simulink model "merged"  (R2024b)
settings: Solver=VariableStepAuto  StartTime=0.0  StopTime=10.0  RelTol=1e-3
libraries: simulink_extras x1
settings Model: PacingRate=0.450000  Creator=Reon Dsouze  LastModifiedBy=Reon Dsouze

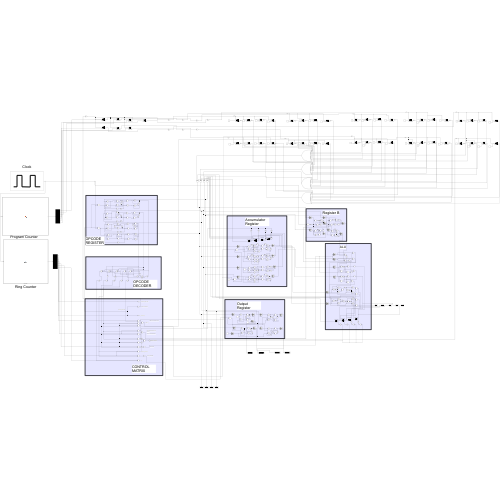
[thumbnail: Simulink's stored preview of the top-level diagram]
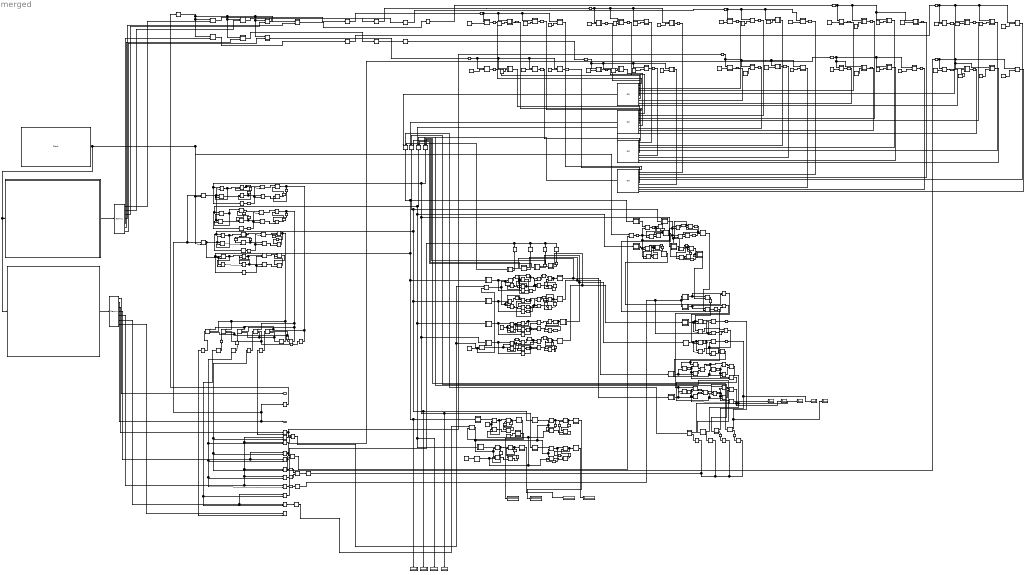
== system merged ==
  note: Clock
  note: Ring Counter
  note: Program Counter
  note: Register B
  note: ALU
  note: Output Register
  note: Accumulator Register
  note: Increment Program Counter
  note: CONTROL MATRIX
  note: enable A reg to data bus
  note: enable subtract
  note: enable sub to data bus from mem
  note: OPCODE DECODER
  note: enable ALU to data bus
  note: enable add to data bus from mem
  note: load A reg
  note: enable load a to data bus from mem
  note: load B reg
  note: halt
  note: Enable mmr to data bus
  note: Opcode reg latches data
  note: grnd mem disp
  note: output reg latches data
  note: OPCODE
      | REGISTER
  AND{,1..9} (10 alike) : Logic  IconShape=distinctive  AllPortsSameDT=off  OutDataTypeStr=boolean
  Clock1 : simulink_extras/Flip Flops/Clock  period=2
  Constant{,1..44} (45 alike) : Constant
  Delay{,1..84} (85 alike) : Delay
  Demux : Demux  Outputs=7
  Demux1 : Demux  Outputs=7
  Display{,1..12} (13 alike) : Display
  NAND{,1..52,54..56,58..60,62..64,66..107,113..120,122..132} (123 alike) : Logic  Operator=NAND  IconShape=distinctive  AllPortsSameDT=off  OutDataTypeStr=boolean
  NAND{53,57,61,65,108..112,121} (10 alike) : Logic  Operator=NAND  Inputs=3  IconShape=distinctive  AllPortsSameDT=off  OutDataTypeStr=boolean
  NOT{,1..72} (73 alike) : Logic  Operator=NOT  IconShape=distinctive  AllPortsSameDT=off  OutDataTypeStr=boolean
  OR : Logic  Operator=OR  IconShape=distinctive  AllPortsSameDT=off  OutDataTypeStr=boolean
  OR1 : Logic  Operator=OR  IconShape=distinctive  AllPortsSameDT=off  OutDataTypeStr=boolean
  OR{2..5} (4 alike) : Logic  Operator=OR  Inputs=3  IconShape=distinctive  AllPortsSameDT=off  OutDataTypeStr=boolean
  OR{6..9} (4 alike) : Logic  Operator=OR  Inputs=10  IconShape=distinctive  AllPortsSameDT=off  OutDataTypeStr=boolean
  Program Counter : MATLAB Function  TreatAsAtomicUnit=on
  Ring Counter : MATLAB Function  TreatAsAtomicUnit=on
  Tri state buffer : Subsystem
      mask Display:
      | % Draw the triangle
      | patch([1 0 1], [0 0.5 1], [0 0 0])  % Left-pointing triangle
  Tri state buffer1 : Subsystem
      mask Display:
      | % Draw the triangle
      | patch([1 0 1], [0 0.5 1], [0 0 0])  % Left-pointing triangle
  Tri state buffer10 : Subsystem
      mask Display:
      | % Draw the triangle
      | patch([1 0 1], [0 0.5 1], [0 0 0])  % Left-pointing triangle
  Tri state buffer11 : Subsystem
      mask Display:
      | % Draw the triangle
      | patch([1 0 1], [0 0.5 1], [0 0 0])  % Left-pointing triangle
  Tri state buffer12 : Subsystem
      mask Display:
      | % Draw the triangle
      | patch([1 0 1], [0 0.5 1], [0 0 0])  % Left-pointing triangle
  Tri state buffer13 : Subsystem
      mask Display:
      | % Draw the triangle
      | patch([1 0 1], [0 0.5 1], [0 0 0])  % Left-pointing triangle
  Tri state buffer14 : Subsystem
      mask Display:
      | % Draw the triangle
      | patch([1 0 1], [0 0.5 1], [0 0 0])  % Left-pointing triangle
  Tri state buffer15 : Subsystem
      mask Display:
      | % Draw the triangle
      | patch([1 0 1], [0 0.5 1], [0 0 0])  % Left-pointing triangle
  Tri state buffer16 : Subsystem
      mask Display:
      | % Draw the triangle
      | patch([1 0 1], [0 0.5 1], [0 0 0])  % Left-pointing triangle
  Tri state buffer17 : Subsystem
      mask Display:
      | % Draw the triangle
      | patch([1 0 1], [0 0.5 1], [0 0 0])  % Left-pointing triangle
  Tri state buffer18 : Subsystem
      mask Display:
      | % Draw the triangle
      | patch([1 0 1], [0 0.5 1], [0 0 0])  % Left-pointing triangle
  Tri state buffer19 : Subsystem
      mask Display:
      | % Draw the triangle
      | patch([1 0 1], [0 0.5 1], [0 0 0])  % Left-pointing triangle
  Tri state buffer2 : Subsystem
      mask Display:
      | % Draw the triangle
      | patch([1 0 1], [0 0.5 1], [0 0 0])  % Left-pointing triangle
  Tri state buffer20 : Subsystem
      mask Display:
      | % Draw the triangle
      | patch([1 0 1], [0 0.5 1], [0 0 0])  % Left-pointing triangle
  Tri state buffer21 : Subsystem
      mask Display:
      | % Draw the triangle
      | patch([1 0 1], [0 0.5 1], [0 0 0])  % Left-pointing triangle
  Tri state buffer22 : Subsystem
      mask Display:
      | % Draw the triangle
      | patch([1 0 1], [0 0.5 1], [0 0 0])  % Left-pointing triangle
  Tri state buffer23 : Subsystem
      mask Display:
      | % Draw the triangle
      | patch([1 0 1], [0 0.5 1], [0 0 0])  % Left-pointing triangle
  Tri state buffer24 : Subsystem
      mask Display:
      | % Draw the triangle
      | patch([1 0 1], [0 0.5 1], [0 0 0])  % Left-pointing triangle
  Tri state buffer25 : Subsystem
      mask Display:
      | % Draw the triangle
      | patch([1 0 1], [0 0.5 1], [0 0 0])  % Left-pointing triangle
  Tri state buffer26 : Subsystem
      mask Display:
      | % Draw the triangle
      | patch([1 0 1], [0 0.5 1], [0 0 0])  % Left-pointing triangle
  Tri state buffer27 : Subsystem
      mask Display:
      | % Draw the triangle
      | patch([1 0 1], [0 0.5 1], [0 0 0])  % Left-pointing triangle
  Tri state buffer28 : Subsystem
      mask Display:
      | % Draw the triangle
      | patch([1 0 1], [0 0.5 1], [0 0 0])  % Left-pointing triangle
  Tri state buffer29 : Subsystem
      mask Display:
      | % Draw the triangle
      | patch([1 0 1], [0 0.5 1], [0 0 0])  % Left-pointing triangle
  Tri state buffer3 : Subsystem
      mask Display:
      | % Draw the triangle
      | patch([1 0 1], [0 0.5 1], [0 0 0])  % Left-pointing triangle
  Tri state buffer30 : Subsystem
      mask Display:
      | % Draw the triangle
      | patch([1 0 1], [0 0.5 1], [0 0 0])  % Left-pointing triangle
  Tri state buffer31 : Subsystem
      mask Display:
      | % Draw the triangle
      | patch([1 0 1], [0 0.5 1], [0 0 0])  % Left-pointing triangle
  Tri state buffer32 : Subsystem
      mask Display:
      | % Draw the triangle
      | patch([1 0 1], [0 0.5 1], [0 0 0])  % Left-pointing triangle
  Tri state buffer33 : Subsystem
      mask Display:
      | % Draw the triangle
      | patch([1 0 1], [0 0.5 1], [0 0 0])  % Left-pointing triangle
  Tri state buffer34 : Subsystem
      mask Display:
      | % Draw the triangle
      | patch([1 0 1], [0 0.5 1], [0 0 0])  % Left-pointing triangle
  Tri state buffer35 : Subsystem
      mask Display:
      | % Draw the triangle
      | patch([1 0 1], [0 0.5 1], [0 0 0])  % Left-pointing triangle
  Tri state buffer36 : Subsystem
      mask Display:
      | % Draw the triangle
      | patch([1 0 1], [0 0.5 1], [0 0 0])  % Left-pointing triangle
  Tri state buffer37 : Subsystem
      mask Display:
      | % Draw the triangle
      | patch([1 0 1], [0 0.5 1], [0 0 0])  % Left-pointing triangle
  Tri state buffer38 : Subsystem
      mask Display:
      | % Draw the triangle
      | patch([1 0 1], [0 0.5 1], [0 0 0])  % Left-pointing triangle
  Tri state buffer39 : Subsystem
      mask Display:
      | % Draw the triangle
      | patch([1 0 1], [0 0.5 1], [0 0 0])  % Left-pointing triangle
  Tri state buffer4 : Subsystem
      mask Display:
      | % Draw the triangle
      | patch([1 0 1], [0 0.5 1], [0 0 0])  % Left-pointing triangle
  Tri state buffer40 : Subsystem
      mask Display:
      | % Draw the triangle
      | patch([1 0 1], [0 0.5 1], [0 0 0])  % Left-pointing triangle
  Tri state buffer41 : Subsystem
      mask Display:
      | % Draw the triangle
      | patch([1 0 1], [0 0.5 1], [0 0 0])  % Left-pointing triangle
  Tri state buffer42 : Subsystem
      mask Display:
      | % Draw the triangle
      | patch([1 0 1], [0 0.5 1], [0 0 0])  % Left-pointing triangle
  Tri state buffer43 : Subsystem
      mask Display:
      | % Draw the triangle
      | patch([1 0 1], [0 0.5 1], [0 0 0])  % Left-pointing triangle
  Tri state buffer44 : Subsystem
      mask Display:
      | % Draw the triangle
      | patch([1 0 1], [0 0.5 1], [0 0 0])  % Left-pointing triangle
  Tri state buffer45 : Subsystem
      mask Display:
      | % Draw the triangle
      | patch([1 0 1], [0 0.5 1], [0 0 0])  % Left-pointing triangle
  Tri state buffer46 : Subsystem
      mask Display:
      | % Draw the triangle
      | patch([1 0 1], [0 0.5 1], [0 0 0])  % Left-pointing triangle
  Tri state buffer47 : Subsystem
      mask Display:
      | % Draw the triangle
      | patch([1 0 1], [0 0.5 1], [0 0 0])  % Left-pointing triangle
  Tri state buffer48 : Subsystem
      mask Display:
      | % Draw the triangle
      | patch([1 0 1], [0 0.5 1], [0 0 0])  % Left-pointing triangle
  Tri state buffer49 : Subsystem
      mask Display:
      | % Draw the triangle
      | patch([1 0 1], [0 0.5 1], [0 0 0])  % Left-pointing triangle
  Tri state buffer5 : Subsystem
      mask Display:
      | % Draw the triangle
      | patch([1 0 1], [0 0.5 1], [0 0 0])  % Left-pointing triangle
  Tri state buffer50 : Subsystem
      mask Display:
      | % Draw the triangle
      | patch([1 0 1], [0 0.5 1], [0 0 0])  % Left-pointing triangle
  Tri state buffer51 : Subsystem
      mask Display:
      | % Draw the triangle
      | patch([1 0 1], [0 0.5 1], [0 0 0])  % Left-pointing triangle
  Tri state buffer52 : Subsystem
      mask Display:
      | % Draw the triangle
      | patch([1 0 1], [0 0.5 1], [0 0 0])  % Left-pointing triangle
  Tri state buffer53 : Subsystem
      mask Display:
      | % Draw the triangle
      | patch([1 0 1], [0 0.5 1], [0 0 0])  % Left-pointing triangle
  Tri state buffer54 : Subsystem
      mask Display:
      | % Draw the triangle
      | patch([1 0 1], [0 0.5 1], [0 0 0])  % Left-pointing triangle
  Tri state buffer55 : Subsystem
      mask Display:
      | % Draw the triangle
      | patch([1 0 1], [0 0.5 1], [0 0 0])  % Left-pointing triangle
  Tri state buffer6 : Subsystem
      mask Display:
      | % Draw the triangle
      | patch([1 0 1], [0 0.5 1], [0 0 0])  % Left-pointing triangle
  Tri state buffer8 : Subsystem
      mask Display:
      | % Draw the triangle
      | patch([1 0 1], [0 0.5 1], [0 0 0])  % Left-pointing triangle
  Tri state buffer9 : Subsystem
      mask Display:
      | % Draw the triangle
      | patch([1 0 1], [0 0.5 1], [0 0 0])  % Left-pointing triangle
  XOR{,1..7} (8 alike) : Logic  Operator=XOR  IconShape=distinctive  AllPortsSameDT=off  OutDataTypeStr=boolean
  buffer : Subsystem
      mask Display: patch([0 1 0], [0 0.5 1], [0.5 0.5 0.5]);  % This draws a triangle
  buffer1 : Subsystem
      mask Display: patch([0 1 0], [0 0.5 1], [0.5 0.5 0.5]);  % This draws a triangle
  buffer10 : Subsystem
      mask Display: patch([0 1 0], [0 0.5 1], [0.5 0.5 0.5]);  % This draws a triangle
  buffer11 : Subsystem
      mask Display: patch([0 1 0], [0 0.5 1], [0.5 0.5 0.5]);  % This draws a triangle
  buffer12 : Subsystem
      mask Display: patch([0 1 0], [0 0.5 1], [0.5 0.5 0.5]);  % This draws a triangle
  buffer13 : Subsystem
      mask Display: patch([0 1 0], [0 0.5 1], [0.5 0.5 0.5]);  % This draws a triangle
  buffer14 : Subsystem
      mask Display: patch([0 1 0], [0 0.5 1], [0.5 0.5 0.5]);  % This draws a triangle
  buffer15 : Subsystem
      mask Display: patch([0 1 0], [0 0.5 1], [0.5 0.5 0.5]);  % This draws a triangle
  buffer16 : Subsystem
      mask Display: patch([0 1 0], [0 0.5 1], [0.5 0.5 0.5]);  % This draws a triangle
  buffer17 : Subsystem
      mask Display: patch([0 1 0], [0 0.5 1], [0.5 0.5 0.5]);  % This draws a triangle
  buffer18 : Subsystem
      mask Display: patch([0 1 0], [0 0.5 1], [0.5 0.5 0.5]);  % This draws a triangle
  buffer19 : Subsystem
      mask Display: patch([0 1 0], [0 0.5 1], [0.5 0.5 0.5]);  % This draws a triangle
  buffer2 : Subsystem
      mask Display: patch([0 1 0], [0 0.5 1], [0.5 0.5 0.5]);  % This draws a triangle
  buffer20 : Subsystem
      mask Display: patch([0 1 0], [0 0.5 1], [0.5 0.5 0.5]);  % This draws a triangle
  buffer21 : Subsystem
      mask Display: patch([0 1 0], [0 0.5 1], [0.5 0.5 0.5]);  % This draws a triangle
  buffer22 : Subsystem
      mask Display: patch([0 1 0], [0 0.5 1], [0.5 0.5 0.5]);  % This draws a triangle
  buffer23 : Subsystem
      mask Display: patch([0 1 0], [0 0.5 1], [0.5 0.5 0.5]);  % This draws a triangle
  buffer24 : Subsystem
      mask Display: patch([0 1 0], [0 0.5 1], [0.5 0.5 0.5]);  % This draws a triangle
  buffer25 : Subsystem
      mask Display: patch([0 1 0], [0 0.5 1], [0.5 0.5 0.5]);  % This draws a triangle
  buffer26 : Subsystem
      mask Display: patch([0 1 0], [0 0.5 1], [0.5 0.5 0.5]);  % This draws a triangle
  buffer27 : Subsystem
      mask Display: patch([0 1 0], [0 0.5 1], [0.5 0.5 0.5]);  % This draws a triangle
  buffer28 : Subsystem
      mask Display: patch([0 1 0], [0 0.5 1], [0.5 0.5 0.5]);  % This draws a triangle
  buffer29 : Subsystem
      mask Display: patch([0 1 0], [0 0.5 1], [0.5 0.5 0.5]);  % This draws a triangle
  buffer3 : Subsystem
      mask Display: patch([0 1 0], [0 0.5 1], [0.5 0.5 0.5]);  % This draws a triangle
  buffer30 : Subsystem
      mask Display: patch([0 1 0], [0 0.5 1], [0.5 0.5 0.5]);  % This draws a triangle
  buffer31 : Subsystem
      mask Display: patch([0 1 0], [0 0.5 1], [0.5 0.5 0.5]);  % This draws a triangle
  buffer4 : Subsystem
      mask Display: patch([0 1 0], [0 0.5 1], [0.5 0.5 0.5]);  % This draws a triangle
  buffer5 : Subsystem
      mask Display: patch([0 1 0], [0 0.5 1], [0.5 0.5 0.5]);  % This draws a triangle
  buffer6 : Subsystem
      mask Display: patch([0 1 0], [0 0.5 1], [0.5 0.5 0.5]);  % This draws a triangle
  buffer7 : Subsystem
      mask Display: patch([0 1 0], [0 0.5 1], [0.5 0.5 0.5]);  % This draws a triangle
  buffer8 : Subsystem
      mask Display: patch([0 1 0], [0 0.5 1], [0.5 0.5 0.5]);  % This draws a triangle
  buffer9 : Subsystem
      mask Display: patch([0 1 0], [0 0.5 1], [0.5 0.5 0.5]);  % This draws a triangle
  Out2 : Outport
  Out3 : Outport  Port=2
  wires:
  buffer15/1(Out1) -> Tri state buffer6/1(In1), buffer5/1(In1)
  NAND80/1 -> NAND79/2
  buffer5/1(Out1) -> NAND9/2, NAND11/2
  NAND76/1 -> NAND75/2
  NAND75/1 -> NAND77/2
  NAND21/1 -> Delay35/1, buffer15/1(In1)
  NAND59/1 -> Delay54/1, buffer27/1(In1)
  NAND7/1 -> Display10/1, Tri state buffer2/1(In1)
  AND1/1 -> Delay78/1
  NAND39/1 -> NAND41/2
  NAND67/1 -> NAND69/2
  Constant2/1 -> NAND50/2, NAND53/1
  XOR5/1 -> Delay67/1
  buffer4/1(Out1) -> NAND/2, NAND2/2
  NAND31/1 -> NAND33/2
  NAND58/1 -> NAND59/1, Delay56/1
  NAND72/1 -> NAND71/2
  NAND63/1 -> Delay57/1, buffer30/1(In1)
  NOT6/1 -> Delay70/1
  NAND45/1 -> Delay19/1, buffer21/1(In1)
  NAND23/1 -> NAND24/2
  NOT7/1 -> Delay66/1
  NOT2/1 -> NAND34/2, NAND35/1
  NAND1/1 -> NAND3/1
  NAND53/1 -> NAND52/2
  buffer1/1(Out1) -> XOR1/1, XOR3/1
  NAND55/1 -> buffer25/1(In1), Delay52/1
  NAND34/1 -> NAND37/1
  Constant1/1 -> AND5/2, AND6/2
  NAND15/1 -> NAND16/2
  buffer14/1(Out1) -> NAND30/1, NOT/1
  buffer7/1(Out1) -> NAND70/1
  NAND6/1 -> NAND7/2
  NAND62/1 -> Delay59/1, NAND63/1
  buffer10/1(Out1) -> XOR3/2
  buffer3/1(Out1) -> AND2/2, XOR6/2
  OR1/1 -> NAND6/2, NAND4/2
  NAND65/1 -> NAND64/2
  OR/1 -> AND3/2, XOR7/2
  buffer20/1(Out1) -> NAND46/1, NOT3/1
  NAND8/1 -> NAND15/2, NAND13/2
  NAND19/1 -> NAND20/2
  NAND2/1 -> NAND3/2
  Constant/1 -> NAND39/1, NAND38/2
  buffer8/1(Out1) -> NAND74/1
  XOR3/1 -> NAND9/1, NAND10/1
  NAND46/1 -> Delay17/1, NAND47/2
  NAND51/1 -> Delay46/1, buffer23/1(In1)
  AND7/1 -> NAND62/2, NAND65/1, NAND57/1, NAND54/2, NAND58/2, NAND61/1
  AND5/1 -> NAND27/1, NAND26/2, NAND31/1, NAND30/2
  XOR/1 -> Delay79/1
  NOT5/1 -> Tri state buffer5/2(In2)
  NAND16/1 -> Display9/1, Tri state buffer3/1(In1)
  NAND27/1 -> NAND29/2
  buffer22/1(Out1) -> NAND50/1
  buffer/1(Out1) -> XOR2/1, XOR/1
  NAND81/1 -> Delay14/1, buffer13/1(In1)
  buffer26/1(Out1) -> NAND58/1
  buffer18/1(Out1) -> NAND38/1, NOT2/1
  AND/1 -> OR/1
  NAND38/1 -> NAND39/2, NAND40/1
  buffer29/1(Out1) -> NAND62/1
  XOR6/1 -> Delay80/1
  NAND35/1 -> NAND36/2
  XOR2/1 -> AND2/1, XOR6/1
  buffer6/1(Out1) -> NAND66/1
  buffer11/1(Out1) -> XOR2/2
  buffer28/1(Out1) -> NAND57/3, NAND53/3, NAND65/3, NAND61/3
  NAND50/1 -> NAND53/2, NAND51/1
  NAND5/1 -> NAND7/1
  XOR7/1 -> Delay71/1
  NAND33/1 -> NAND32/2, NAND19/2
  buffer19/1(Out1) -> Tri state buffer4/1(In1), buffer3/1(In1)
  NAND54/1 -> Delay53/1, NAND55/1
  NAND25/1 -> Delay31/1, buffer17/1(In1)
  buffer13/1(Out1) -> XOR/2
  buffer9/1(Out1) -> NAND78/1
  buffer24/1(Out1) -> NAND54/1
  AND6/1 -> NAND46/2, NAND47/1
  AND4/1 -> Delay21/1
  NOT3/1 -> NAND42/2, NAND43/1
  NAND47/1 -> NAND49/2
  buffer16/1(Out1) -> NAND26/1, NOT1/1
  NOT4/1 -> Tri state buffer6/2(In2)
  NAND14/1 -> NAND16/1
  NAND40/1 -> NAND41/1, NAND34/1
  NAND57/1 -> NAND56/2
  NAND43/1 -> NAND44/2
  AND3/1 -> OR1/2
  AND2/1 -> OR1/1
  buffer31/1(Out1) -> AND7/2
  buffer21/1(Out1) -> Tri state buffer52/1(In1), buffer2/1(In1)
  NAND68/1 -> NAND67/2
  buffer2/1(Out1) -> AND/2, XOR4/2
  buffer12/1(Out1) -> XOR1/2
  XOR4/1 -> Delay77/1
  NAND61/1 -> NAND60/2
  buffer17/1(Out1) -> Tri state buffer5/1(In1), buffer4/1(In1)
  NAND105/1 -> Delay/1, NAND127/1
  Demux1/3 -> NAND113/1
  Demux1/5 -> NAND126/1, NAND125/1, NAND120/1, NAND114/1, NAND115/1
  Demux1/1 -> Out3/1
  NOT22/1 -> NAND113/2
  NAND109/1 -> Delay76/1
  NAND103/1 -> NAND107/1
  NOT10/1 -> Delay74/1
  NAND108/1 -> NOT18/1
  NAND85/1 -> Delay4/1, NAND87/1
  NAND110/1 -> Delay84/1
  NAND100/1 -> NAND102/2
  NAND90/1 -> NAND91/2, NAND92/1
  OR4/1 -> NOT9/1, NAND131/1, buffer8/1(In1), Display6/1, buffer26/1(In1), buffer18/1(In1)
  NAND94/1 -> Delay1/1, NAND116/1
  NAND101/1 -> NAND102/1, NAND103/1
  NAND91/1 -> NAND93/2
  NOT9/1 -> Delay69/1
  NAND114/1 -> NAND121/2
  OR2/1 -> buffer6/1(In1), NOT17/1, NAND99/1, Display4/1, buffer22/1(In1), buffer14/1(In1)
  NOT18/1 -> NAND119/2
  NAND86/1 -> NAND89/1
  NOT17/1 -> NAND104/2, NAND103/2
  NAND130/1 -> Delay3/1, NOT11/1, NAND108/1, NAND110/1, NAND112/1
  NAND115/1 -> Delay81/1
  AND9/1 -> NAND91/1, NAND90/2, NAND100/1, NAND99/2
  NAND89/1 -> Delay7/1, NAND110/2, NOT10/1, NAND111/1
  NAND104/1 -> NAND106/2
  NAND123/1 -> NOT72/1, NAND124/2
  Ring Counter/1(y) -> Demux1/1
  Demux1/7 -> NAND119/1
  NAND128/1 -> NOT12/1
  NAND95/1 -> NAND98/1
  NOT11/1 -> Delay75/1
  Demux1/4 -> NAND122/1, NAND123/1
  NAND132/1 -> NAND85/2
  NOT23/1 -> NAND110/3, NAND111/3, NAND112/3
  NAND82/1 -> NAND83/2, NAND94/1
  Demux1/2 -> Out2/1, AND9/1, AND8/1, NOT15/1
  NOT8/1 -> Delay65/1
  NAND112/1 -> NOT22/1
  NAND107/1 -> NAND106/1
  NAND83/1 -> NAND105/2
  NAND98/1 -> Delay10/1, NAND108/2, NAND109/1, NOT23/1
  NOT20/1 -> NAND115/2, NAND126/2, NAND123/2, NAND120/2
  NAND93/1 -> Delay8/1, NAND96/1
  NAND84/1 -> Delay5/1, NAND86/1
  NAND92/1 -> Delay9/1, NAND95/1
  Demux1/6 -> NAND117/1, NAND118/1
  OR3/1 -> buffer7/1(In1), Display5/1, buffer24/1(In1), buffer16/1(In1), NOT16/1, NAND90/1
  NAND122/1 -> NOT71/1, NAND124/1
  NAND102/1 -> NAND104/1, NAND101/2
  Clock1/1 -> AND4/1, AND9/2, AND8/2, Ring Counter/1(clk), Program Counter/1(clk)
  NOT19/1 -> NAND118/2, NAND117/2
  NAND113/1 -> NOT70/1, NAND121/1
  NOT21/1 -> NAND125/2, NAND122/2, NAND114/2
  NAND99/1 -> NAND100/2, NAND101/1
  NOT16/1 -> Delay73/1
  NAND96/1 -> NAND97/2
  Program Counter/1(y) -> Demux/1
  NAND118/1 -> NOT14/1
  OR5/1 -> buffer9/1(In1), Display7/1, buffer29/1(In1), buffer20/1(In1), NOT8/1, NAND82/1
  NAND126/1 -> Delay82/1
  NAND120/1 -> NAND121/3
  AND8/1 -> NAND131/2, NAND132/1, NAND83/1, NAND82/2
  NAND125/1 -> Delay83/1
  NAND111/1 -> NOT21/1
  NAND127/1 -> NAND129/2
  NAND106/1 -> NAND107/2
  NAND116/1 -> NAND130/1
  NAND131/1 -> NAND132/2, NAND84/1
  NAND87/1 -> NAND88/2
  NOT24/1 -> Tri state buffer3/2(In2)
  NOT25/1 -> Tri state buffer2/2(In2)
  NOT26/1 -> Delay72/1
  NOT27/1 -> Delay68/1
  NOT12/1 -> NOT25/1, NOT26/1, NOT27/1, NOT24/1
  NOT13/1 -> XOR5/2, AND1/2, buffer1/1(In1), buffer/1(In1)
  NOT14/1 -> AND7/1
  NAND121/1 -> AND6/1, AND5/1
  Constant3/1 -> buffer28/1(In1)
  Tri state buffer3/1(Out1) -> OR2/2
  Tri state buffer2/1(Out1) -> OR3/2
  Tri state buffer1/1(Out1) -> OR4/2
  Tri state buffer/1(Out1) -> OR5/2
  Tri state buffer6/1(Out1) -> OR2/3
  Tri state buffer5/1(Out1) -> OR3/3
  Tri state buffer4/1(Out1) -> OR4/3
  Tri state buffer52/1(Out1) -> OR5/3
  Tri state buffer13/1(Out1) -> OR8/2
  Tri state buffer38/1(Out1) -> OR8/9
  Tri state buffer43/1(Out1) -> OR9/8
  Tri state buffer34/1(Out1) -> OR9/7
  Tri state buffer31/1(Out1) -> OR7/7
  Tri state buffer47/1(Out1) -> OR9/10
  Tri state buffer19/1(Out1) -> OR8/4
  Tri state buffer17/1(Out1) -> OR8/3
  Tri state buffer25/1(Out1) -> OR8/5
  Tri state buffer45/1(Out1) -> OR8/10
  Tri state buffer27/1(Out1) -> OR9/5
  Tri state buffer28/1(Out1) -> OR7/6
  Tri state buffer42/1(Out1) -> NOT56/1
  Tri state buffer39/1(Out1) -> NOT53/1
  NOT36/1 -> Tri state buffer20/1(In1), Tri state buffer18/1(In1), Tri state buffer21/1(In1), Tri state buffer19/1(In1)
  Tri state buffer16/1(Out1) -> NOT43/1
  NOT31/1 -> Tri state buffer14/1(In1), Tri state buffer12/1(In1), Tri state buffer15/1(In1), Tri state buffer13/1(In1)
  Tri state buffer51/1(Out1) -> NOT29/1
  Tri state buffer54/1(Out1) -> NOT55/1
  Tri state buffer32/1(Out1) -> NOT49/1
  Tri state buffer33/1(Out1) -> NOT50/1
  NOT28/1 -> Tri state buffer54/1(In1), Tri state buffer8/1(In1), Tri state buffer50/1(In1), Tri state buffer30/1(In1), Tri state buffer9/1(In1), Tri state buffer51/1(In1), Tri state buffer41/1(In1)
  Tri state buffer22/1(Out1) -> NOT42/1
  Tri state buffer48/1(Out1) -> NOT47/1
  Tri state buffer36/1(Out1) -> NOT51/1
  Tri state buffer23/1(Out1) -> NOT37/1
  NOT65/1 -> Tri state buffer33/1(In1), Tri state buffer31/1(In1), Tri state buffer34/1(In1), Tri state buffer32/1(In1)
  Tri state buffer18/1(Out1) -> NOT41/1
  Tri state buffer35/1(Out1) -> NOT57/1
  NOT32/1 -> Tri state buffer22/1(In1), Tri state buffer16/1(In1), Tri state buffer23/1(In1), Tri state buffer17/1(In1)
  Tri state buffer30/1(Out1) -> NOT39/1
  NOT63/1 -> NOT62/1
  Tri state buffer50/1(Out1) -> NOT48/1
  Tri state buffer44/1(Out1) -> NOT59/1
  Tri state buffer10/1(Out1) -> NOT69/1
  Tri state buffer41/1(Out1) -> NOT63/1
  Tri state buffer24/1(Out1) -> NOT45/1
  NOT66/1 -> NOT64/1
  Tri state buffer9/1(Out1) -> NOT66/1
  Tri state buffer14/1(Out1) -> NOT34/1
  Tri state buffer12/1(Out1) -> NOT35/1
  Tri state buffer21/1(Out1) -> NOT38/1
  NOT39/1 -> NOT31/1
  Tri state buffer8/1(Out1) -> NOT67/1
  Tri state buffer46/1(Out1) -> NOT58/1
  NOT61/1 -> Tri state buffer49/1(In1), Tri state buffer10/1(In1), Tri state buffer53/1(In1), Tri state buffer11/1(In1)
  Tri state buffer11/1(Out1) -> NOT30/1
  Tri state buffer37/1(Out1) -> NOT54/1
  Tri state buffer55/1(Out1) -> NOT60/1
  NOT29/1 -> NOT61/1
  Tri state buffer49/1(Out1) -> NOT68/1
  NOT67/1 -> NOT65/1
  NOT62/1 -> Tri state buffer26/1(In1), Tri state buffer24/1(In1), Tri state buffer27/1(In1), Tri state buffer25/1(In1)
  NOT48/1 -> NOT32/1
  Tri state buffer29/1(Out1) -> NOT46/1
  Tri state buffer40/1(Out1) -> NOT52/1
  NOT64/1 -> Tri state buffer55/1(In1), Tri state buffer28/1(In1), Tri state buffer48/1(In1), Tri state buffer29/1(In1)
  Tri state buffer15/1(Out1) -> NOT33/1
  NOT55/1 -> NOT36/1
  NOT15/1 -> NOT28/1
  Demux/1 -> Tri state buffer51/2(In2)
  Demux/2 -> Tri state buffer30/2(In2)
  Demux/3 -> Tri state buffer50/2(In2)
  Demux/4 -> Tri state buffer54/2(In2)
  Demux/5 -> Tri state buffer41/2(In2)
  Demux/6 -> Tri state buffer9/2(In2)
  Demux/7 -> Tri state buffer8/2(In2)
  NOT70/1 -> Tri state buffer42/1(In1), Tri state buffer35/1(In1), Tri state buffer43/1(In1), Tri state buffer36/1(In1)
  NOT71/1 -> Tri state buffer40/1(In1), Tri state buffer38/1(In1), Tri state buffer37/1(In1), Tri state buffer39/1(In1)
  NOT72/1 -> Tri state buffer46/1(In1), Tri state buffer47/1(In1), Tri state buffer45/1(In1), Tri state buffer44/1(In1)
  Tri state buffer26/1(Out1) -> NOT44/1
  NOT68/1 -> OR6/1
  NOT69/1 -> OR7/1
  NOT34/1 -> OR6/2
  NOT42/1 -> OR6/3
  Tri state buffer20/1(Out1) -> NOT40/1
  NOT40/1 -> OR6/4
  NOT44/1 -> OR6/5
  NOT60/1 -> OR6/6
  NOT50/1 -> OR6/7
  NOT56/1 -> OR6/8
  NOT53/1 -> OR6/9
  NOT58/1 -> OR6/10
  OR6/1 -> OR2/1
  OR7/1 -> OR3/1
  OR8/1 -> OR4/1
  OR9/1 -> OR5/1
  NOT35/1 -> OR7/2
  NOT43/1 -> OR7/3
  NOT41/1 -> OR7/4
  NOT45/1 -> OR7/5
  NOT57/1 -> OR7/8
  NOT54/1 -> OR7/9
  NOT59/1 -> OR7/10
  NOT30/1 -> OR8/1
  NOT46/1 -> OR8/6
  NOT49/1 -> OR8/7
  NOT51/1 -> OR8/8
  Tri state buffer53/1(Out1) -> OR9/1
  NOT33/1 -> OR9/2
  NOT37/1 -> OR9/3
  NOT38/1 -> OR9/4
  NOT47/1 -> OR9/6
  NOT52/1 -> OR9/9
  Constant4/1 -> Tri state buffer49/2(In2)
  Constant5/1 -> Tri state buffer10/2(In2)
  Constant6/1 -> Tri state buffer11/2(In2)
  Constant7/1 -> Tri state buffer53/2(In2)
  Constant8/1 -> Tri state buffer14/2(In2)
  Constant9/1 -> Tri state buffer12/2(In2)
  Constant10/1 -> Tri state buffer13/2(In2)
  Constant11/1 -> Tri state buffer15/2(In2)
  Constant12/1 -> Tri state buffer22/2(In2)
  Constant13/1 -> Tri state buffer16/2(In2)
  Constant14/1 -> Tri state buffer17/2(In2)
  Constant15/1 -> Tri state buffer23/2(In2)
  Constant16/1 -> Tri state buffer20/2(In2)
  Constant17/1 -> Tri state buffer18/2(In2)
  Constant18/1 -> Tri state buffer19/2(In2)
  Constant19/1 -> Tri state buffer21/2(In2)
  Constant20/1 -> Tri state buffer26/2(In2)
  Constant21/1 -> Tri state buffer24/2(In2)
  Constant22/1 -> Tri state buffer25/2(In2)
  Constant23/1 -> Tri state buffer27/2(In2)
  Constant24/1 -> Tri state buffer55/2(In2)
  Constant25/1 -> Tri state buffer28/2(In2)
  Constant26/1 -> Tri state buffer29/2(In2)
  Constant27/1 -> Tri state buffer48/2(In2)
  Constant28/1 -> Tri state buffer33/2(In2)
  Constant29/1 -> Tri state buffer31/2(In2)
  Constant30/1 -> Tri state buffer32/2(In2)
  Constant31/1 -> Tri state buffer34/2(In2)
  Constant32/1 -> Tri state buffer42/2(In2)
  Constant33/1 -> Tri state buffer35/2(In2)
  Constant34/1 -> Tri state buffer36/2(In2)
  Constant35/1 -> Tri state buffer43/2(In2)
  Constant36/1 -> Tri state buffer39/2(In2)
  Constant37/1 -> Tri state buffer37/2(In2)
  Constant38/1 -> Tri state buffer38/2(In2)
  Constant39/1 -> Tri state buffer40/2(In2)
  Constant40/1 -> Tri state buffer46/2(In2)
  Constant41/1 -> Tri state buffer44/2(In2)
  Constant42/1 -> Tri state buffer45/2(In2)
  Constant43/1 -> Tri state buffer47/2(In2)
  NAND124/1 -> AND4/2
  NAND117/1 -> NOT4/1, NOT5/1, NOT6/1, NOT7/1
  buffer23/1(Out1) -> Display/1
  buffer25/1(Out1) -> Display1/1
  buffer27/1(Out1) -> Display2/1
  buffer30/1(Out1) -> Display3/1
  Delay/1 -> NAND94/2
  Delay1/1 -> NAND105/1
  NAND129/1 -> Delay2/1
  Delay2/1 -> NAND130/2
  Delay3/1 -> NAND129/1
  Delay4/1 -> NAND84/2
  Delay5/1 -> NAND85/1
  Delay6/1 -> NAND89/2
  NAND88/1 -> Delay6/1
  Delay7/1 -> NAND88/1
  Delay8/1 -> NAND92/2
  Delay9/1 -> NAND93/1
  Delay10/1 -> NAND97/1
  Delay11/1 -> NAND98/2
  NAND97/1 -> Delay11/1
  Delay13/1 -> NAND81/2
  NAND79/1 -> Delay13/1
  Delay14/1 -> NAND79/1
  Delay15/1 -> NAND45/1
  NAND42/1 -> Delay15/1
  Delay16/1 -> NAND49/1, NAND42/1
  Delay17/1 -> NAND48/1
  NAND44/1 -> Delay18/1
  Delay18/1 -> NAND45/2
  Delay19/1 -> NAND44/1
  NAND78/1 -> Delay12/1
  Delay12/1 -> NAND80/2, NAND81/1
  Delay20/1 -> NAND76/2, NAND77/1
  NAND74/1 -> Delay20/1
  Delay21/1 -> NAND80/1, NAND78/2, NAND72/1, NAND70/2, NAND76/1, NAND74/2, NAND66/2, NAND68/1
  Delay22/1 -> NAND75/1
  NAND77/1 -> Delay22/1
  NAND41/1 -> Delay23/1
  Delay23/1 -> NAND40/2, NAND35/2
  NAND36/1 -> Delay24/1
  Delay24/1 -> NAND37/2
  NAND37/1 -> Delay25/1
  Delay25/1 -> NAND36/1, buffer19/1(In1)
  NAND/1 -> Delay26/1
  Delay26/1 -> NAND8/2, NAND2/1, NAND1/2
  XOR1/1 -> Delay27/1
  Delay27/1 -> NAND/1, NAND1/1
  NAND29/1 -> Delay28/1
  Delay28/1 -> NAND28/2, NAND23/2
  NAND4/1 -> Delay29/1
  Delay29/1 -> NAND8/1, NAND6/1, NAND5/2
  NAND24/1 -> Delay30/1
  Delay30/1 -> NAND25/2
  Delay31/1 -> NAND24/1
  NAND28/1 -> Delay32/1
  Delay32/1 -> NAND29/1, NAND22/1
  NAND26/1 -> Delay33/1
  Delay33/1 -> NAND28/1, NAND27/2
  NAND20/1 -> Delay34/1
  Delay34/1 -> NAND21/2
  Delay35/1 -> NAND20/1
  NAND32/1 -> Delay36/1
  Delay36/1 -> NAND33/1, NAND18/1
  NAND30/1 -> Delay37/1
  Delay37/1 -> NAND31/2, NAND32/1
  NAND18/1 -> Delay38/1
  Delay38/1 -> NAND21/1
  NOT/1 -> Delay39/1
  Delay39/1 -> NAND19/1, NAND18/2
  NAND13/1 -> Delay40/1
  Delay40/1 -> NAND14/2, NAND17/1, NAND15/1
  Delay41/1 -> NAND14/1, NAND13/1
  NAND12/1 -> Delay41/1
  Delay43/1 -> NAND12/2
  Delay42/1 -> NAND12/1
  NAND10/1 -> Delay42/1
  NAND11/1 -> Delay43/1
  NAND9/1 -> Delay44/1
  Delay44/1 -> NAND17/2, NAND11/1, NAND10/2
  Delay45/1 -> NAND68/2, NAND69/1
  NAND66/1 -> Delay45/1
  Delay46/1 -> NAND52/1
  Delay47/1 -> NAND51/2
  NAND52/1 -> Delay47/1
  NAND22/1 -> Delay48/1
  Delay48/1 -> NAND25/1
  NOT1/1 -> Delay49/1
  Delay49/1 -> NAND22/2, NAND23/1
  NAND3/1 -> Delay50/1
  Delay50/1 -> NAND5/1, NAND4/1
  Delay51/1 -> NAND55/2
  NAND56/1 -> Delay51/1
  Delay52/1 -> NAND56/1
  Delay53/1 -> NAND57/2
  Delay54/1 -> NAND60/1
  NAND60/1 -> Delay55/1
  Delay55/1 -> NAND59/2
  Delay56/1 -> NAND61/2
  Delay57/1 -> NAND64/1
  NAND64/1 -> Delay58/1
  Delay58/1 -> NAND63/2
  Delay59/1 -> NAND65/2
  NAND69/1 -> Delay60/1
  Delay60/1 -> buffer10/1(In1), NAND67/1
  NAND49/1 -> Delay61/1
  Delay61/1 -> NAND48/2, NAND43/2
  NAND48/1 -> Delay16/1
  NAND70/1 -> Delay62/1
  Delay62/1 -> NAND72/2, NAND73/1
  NAND73/1 -> Delay63/1
  Delay63/1 -> buffer12/1(In1), NAND71/1
  NAND71/1 -> Delay64/1
  Delay64/1 -> NAND73/2
  Constant44/1 -> buffer31/1(In1)
  Delay65/1 -> NAND127/2, NAND116/2
  Delay66/1 -> Tri state buffer52/2(In2)
  Delay67/1 -> Display12/1, Tri state buffer/1(In1)
  Delay68/1 -> Tri state buffer/2(In2)
  Delay69/1 -> NAND87/2, NAND86/2
  Delay70/1 -> Tri state buffer4/2(In2)
  Delay71/1 -> Tri state buffer1/1(In1), Display11/1
  Delay72/1 -> Tri state buffer1/2(In2)
  Delay73/1 -> NAND96/2, NAND95/2
  Delay74/1 -> NAND108/3, NAND109/3, NAND112/2
  Delay75/1 -> NAND109/2, NAND111/2
  Delay76/1 -> NOT19/1
  Delay77/1 -> XOR5/1, AND1/1
  Delay78/1 -> OR/2
  Delay79/1 -> AND/1, XOR4/1
  Delay80/1 -> XOR7/1, AND3/1
  Delay81/1 -> NOT13/1
  Delay82/1 -> NAND128/2
  Delay83/1 -> NAND128/1
  Delay84/1 -> NOT20/1
  NAND17/1 -> Display8/1

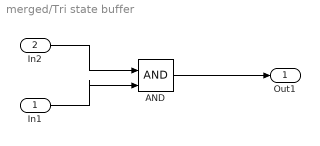
== system merged/Tri state buffer ==
  In1 : Inport
  In2 : Inport  Port=2
  AND : Logic  IconShape=distinctive  AllPortsSameDT=off  OutDataTypeStr=boolean
  Out1 : Outport
  wires:
  In1/1 -> AND/2
  In2/1 -> AND/1
  AND/1 -> Out1/1

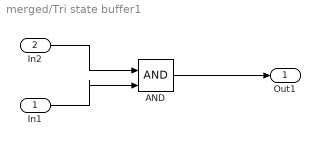
== system merged/Tri state buffer1 ==
  In1 : Inport
  In2 : Inport  Port=2
  AND : Logic  IconShape=distinctive  AllPortsSameDT=off  OutDataTypeStr=boolean
  Out1 : Outport
  wires:
  AND/1 -> Out1/1
  In2/1 -> AND/1
  In1/1 -> AND/2

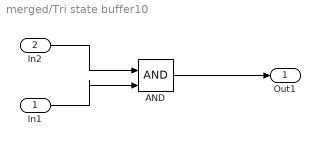
== system merged/Tri state buffer10 ==
  In1 : Inport
  In2 : Inport  Port=2
  AND : Logic  IconShape=distinctive  AllPortsSameDT=off  OutDataTypeStr=boolean
  Out1 : Outport
  wires:
  AND/1 -> Out1/1
  In2/1 -> AND/1
  In1/1 -> AND/2

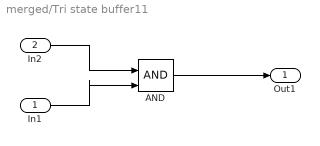
== system merged/Tri state buffer11 ==
  In1 : Inport
  In2 : Inport  Port=2
  AND : Logic  IconShape=distinctive  AllPortsSameDT=off  OutDataTypeStr=boolean
  Out1 : Outport
  wires:
  In1/1 -> AND/2
  In2/1 -> AND/1
  AND/1 -> Out1/1

== system merged/Tri state buffer12 ==
  In1 : Inport
  In2 : Inport  Port=2
  AND : Logic  IconShape=distinctive  AllPortsSameDT=off  OutDataTypeStr=boolean
  Out1 : Outport
  wires:
  In1/1 -> AND/2
  In2/1 -> AND/1
  AND/1 -> Out1/1

== system merged/Tri state buffer13 ==
  In1 : Inport
  In2 : Inport  Port=2
  AND : Logic  IconShape=distinctive  AllPortsSameDT=off  OutDataTypeStr=boolean
  Out1 : Outport
  wires:
  AND/1 -> Out1/1
  In2/1 -> AND/1
  In1/1 -> AND/2

== system merged/Tri state buffer14 ==
  In1 : Inport
  In2 : Inport  Port=2
  AND : Logic  IconShape=distinctive  AllPortsSameDT=off  OutDataTypeStr=boolean
  Out1 : Outport
  wires:
  AND/1 -> Out1/1
  In2/1 -> AND/1
  In1/1 -> AND/2

== system merged/Tri state buffer15 ==
  In1 : Inport
  In2 : Inport  Port=2
  AND : Logic  IconShape=distinctive  AllPortsSameDT=off  OutDataTypeStr=boolean
  Out1 : Outport
  wires:
  In1/1 -> AND/2
  In2/1 -> AND/1
  AND/1 -> Out1/1

== system merged/Tri state buffer16 ==
  In1 : Inport
  In2 : Inport  Port=2
  AND : Logic  IconShape=distinctive  AllPortsSameDT=off  OutDataTypeStr=boolean
  Out1 : Outport
  wires:
  AND/1 -> Out1/1
  In2/1 -> AND/1
  In1/1 -> AND/2

== system merged/Tri state buffer17 ==
  In1 : Inport
  In2 : Inport  Port=2
  AND : Logic  IconShape=distinctive  AllPortsSameDT=off  OutDataTypeStr=boolean
  Out1 : Outport
  wires:
  In1/1 -> AND/2
  In2/1 -> AND/1
  AND/1 -> Out1/1

== system merged/Tri state buffer18 ==
  In1 : Inport
  In2 : Inport  Port=2
  AND : Logic  IconShape=distinctive  AllPortsSameDT=off  OutDataTypeStr=boolean
  Out1 : Outport
  wires:
  In1/1 -> AND/2
  In2/1 -> AND/1
  AND/1 -> Out1/1

== system merged/Tri state buffer19 ==
  In1 : Inport
  In2 : Inport  Port=2
  AND : Logic  IconShape=distinctive  AllPortsSameDT=off  OutDataTypeStr=boolean
  Out1 : Outport
  wires:
  AND/1 -> Out1/1
  In2/1 -> AND/1
  In1/1 -> AND/2

== system merged/Tri state buffer2 ==
  In1 : Inport
  In2 : Inport  Port=2
  AND : Logic  IconShape=distinctive  AllPortsSameDT=off  OutDataTypeStr=boolean
  Out1 : Outport
  wires:
  In1/1 -> AND/2
  In2/1 -> AND/1
  AND/1 -> Out1/1

== system merged/Tri state buffer20 ==
  In1 : Inport
  In2 : Inport  Port=2
  AND : Logic  IconShape=distinctive  AllPortsSameDT=off  OutDataTypeStr=boolean
  Out1 : Outport
  wires:
  AND/1 -> Out1/1
  In2/1 -> AND/1
  In1/1 -> AND/2

== system merged/Tri state buffer21 ==
  In1 : Inport
  In2 : Inport  Port=2
  AND : Logic  IconShape=distinctive  AllPortsSameDT=off  OutDataTypeStr=boolean
  Out1 : Outport
  wires:
  In1/1 -> AND/2
  In2/1 -> AND/1
  AND/1 -> Out1/1

== system merged/Tri state buffer22 ==
  In1 : Inport
  In2 : Inport  Port=2
  AND : Logic  IconShape=distinctive  AllPortsSameDT=off  OutDataTypeStr=boolean
  Out1 : Outport
  wires:
  In1/1 -> AND/2
  In2/1 -> AND/1
  AND/1 -> Out1/1

== system merged/Tri state buffer23 ==
  In1 : Inport
  In2 : Inport  Port=2
  AND : Logic  IconShape=distinctive  AllPortsSameDT=off  OutDataTypeStr=boolean
  Out1 : Outport
  wires:
  AND/1 -> Out1/1
  In2/1 -> AND/1
  In1/1 -> AND/2

== system merged/Tri state buffer24 ==
  In1 : Inport
  In2 : Inport  Port=2
  AND : Logic  IconShape=distinctive  AllPortsSameDT=off  OutDataTypeStr=boolean
  Out1 : Outport
  wires:
  AND/1 -> Out1/1
  In2/1 -> AND/1
  In1/1 -> AND/2

== system merged/Tri state buffer25 ==
  In1 : Inport
  In2 : Inport  Port=2
  AND : Logic  IconShape=distinctive  AllPortsSameDT=off  OutDataTypeStr=boolean
  Out1 : Outport
  wires:
  In1/1 -> AND/2
  In2/1 -> AND/1
  AND/1 -> Out1/1

== system merged/Tri state buffer26 ==
  In1 : Inport
  In2 : Inport  Port=2
  AND : Logic  IconShape=distinctive  AllPortsSameDT=off  OutDataTypeStr=boolean
  Out1 : Outport
  wires:
  In1/1 -> AND/2
  In2/1 -> AND/1
  AND/1 -> Out1/1

== system merged/Tri state buffer27 ==
  In1 : Inport
  In2 : Inport  Port=2
  AND : Logic  IconShape=distinctive  AllPortsSameDT=off  OutDataTypeStr=boolean
  Out1 : Outport
  wires:
  AND/1 -> Out1/1
  In2/1 -> AND/1
  In1/1 -> AND/2

== system merged/Tri state buffer28 ==
  In1 : Inport
  In2 : Inport  Port=2
  AND : Logic  IconShape=distinctive  AllPortsSameDT=off  OutDataTypeStr=boolean
  Out1 : Outport
  wires:
  In1/1 -> AND/2
  In2/1 -> AND/1
  AND/1 -> Out1/1

== system merged/Tri state buffer29 ==
  In1 : Inport
  In2 : Inport  Port=2
  AND : Logic  IconShape=distinctive  AllPortsSameDT=off  OutDataTypeStr=boolean
  Out1 : Outport
  wires:
  AND/1 -> Out1/1
  In2/1 -> AND/1
  In1/1 -> AND/2

== system merged/Tri state buffer3 ==
  In1 : Inport
  In2 : Inport  Port=2
  AND : Logic  IconShape=distinctive  AllPortsSameDT=off  OutDataTypeStr=boolean
  Out1 : Outport
  wires:
  AND/1 -> Out1/1
  In2/1 -> AND/1
  In1/1 -> AND/2

== system merged/Tri state buffer30 ==
  In1 : Inport
  In2 : Inport  Port=2
  AND : Logic  IconShape=distinctive  AllPortsSameDT=off  OutDataTypeStr=boolean
  Out1 : Outport
  wires:
  AND/1 -> Out1/1
  In2/1 -> AND/1
  In1/1 -> AND/2

== system merged/Tri state buffer31 ==
  In1 : Inport
  In2 : Inport  Port=2
  AND : Logic  IconShape=distinctive  AllPortsSameDT=off  OutDataTypeStr=boolean
  Out1 : Outport
  wires:
  In1/1 -> AND/2
  In2/1 -> AND/1
  AND/1 -> Out1/1

== system merged/Tri state buffer32 ==
  In1 : Inport
  In2 : Inport  Port=2
  AND : Logic  IconShape=distinctive  AllPortsSameDT=off  OutDataTypeStr=boolean
  Out1 : Outport
  wires:
  AND/1 -> Out1/1
  In2/1 -> AND/1
  In1/1 -> AND/2

== system merged/Tri state buffer33 ==
  In1 : Inport
  In2 : Inport  Port=2
  AND : Logic  IconShape=distinctive  AllPortsSameDT=off  OutDataTypeStr=boolean
  Out1 : Outport
  wires:
  AND/1 -> Out1/1
  In2/1 -> AND/1
  In1/1 -> AND/2

== system merged/Tri state buffer34 ==
  In1 : Inport
  In2 : Inport  Port=2
  AND : Logic  IconShape=distinctive  AllPortsSameDT=off  OutDataTypeStr=boolean
  Out1 : Outport
  wires:
  In1/1 -> AND/2
  In2/1 -> AND/1
  AND/1 -> Out1/1

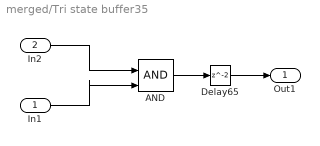
== system merged/Tri state buffer35 ==
  In1 : Inport
  In2 : Inport  Port=2
  AND : Logic  IconShape=distinctive  AllPortsSameDT=off  OutDataTypeStr=boolean
  Delay65 : Delay
  Out1 : Outport
  wires:
  In1/1 -> AND/2
  In2/1 -> AND/1
  AND/1 -> Delay65/1
  Delay65/1 -> Out1/1

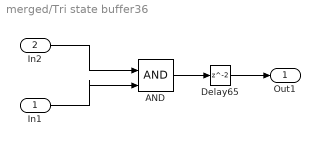
== system merged/Tri state buffer36 ==
  In1 : Inport
  In2 : Inport  Port=2
  AND : Logic  IconShape=distinctive  AllPortsSameDT=off  OutDataTypeStr=boolean
  Delay65 : Delay
  Out1 : Outport
  wires:
  AND/1 -> Delay65/1
  In2/1 -> AND/1
  In1/1 -> AND/2
  Delay65/1 -> Out1/1

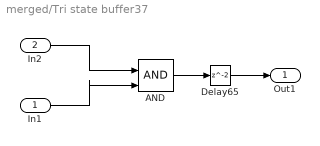
== system merged/Tri state buffer37 ==
  In1 : Inport
  In2 : Inport  Port=2
  AND : Logic  IconShape=distinctive  AllPortsSameDT=off  OutDataTypeStr=boolean
  Delay65 : Delay
  Out1 : Outport
  wires:
  In1/1 -> AND/2
  In2/1 -> AND/1
  AND/1 -> Delay65/1
  Delay65/1 -> Out1/1

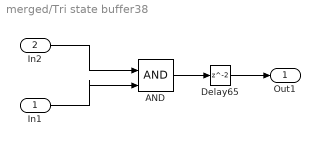
== system merged/Tri state buffer38 ==
  In1 : Inport
  In2 : Inport  Port=2
  AND : Logic  IconShape=distinctive  AllPortsSameDT=off  OutDataTypeStr=boolean
  Delay65 : Delay
  Out1 : Outport
  wires:
  AND/1 -> Delay65/1
  In2/1 -> AND/1
  In1/1 -> AND/2
  Delay65/1 -> Out1/1

== system merged/Tri state buffer39 ==
  In1 : Inport
  In2 : Inport  Port=2
  AND : Logic  IconShape=distinctive  AllPortsSameDT=off  OutDataTypeStr=boolean
  Out1 : Outport
  wires:
  AND/1 -> Out1/1
  In2/1 -> AND/1
  In1/1 -> AND/2

== system merged/Tri state buffer4 ==
  In1 : Inport
  In2 : Inport  Port=2
  AND : Logic  IconShape=distinctive  AllPortsSameDT=off  OutDataTypeStr=boolean
  Out1 : Outport
  wires:
  In1/1 -> AND/2
  In2/1 -> AND/1
  AND/1 -> Out1/1

== system merged/Tri state buffer40 ==
  In1 : Inport
  In2 : Inport  Port=2
  AND : Logic  IconShape=distinctive  AllPortsSameDT=off  OutDataTypeStr=boolean
  Out1 : Outport
  wires:
  In1/1 -> AND/2
  In2/1 -> AND/1
  AND/1 -> Out1/1

== system merged/Tri state buffer41 ==
  In1 : Inport
  In2 : Inport  Port=2
  AND : Logic  IconShape=distinctive  AllPortsSameDT=off  OutDataTypeStr=boolean
  Out1 : Outport
  wires:
  AND/1 -> Out1/1
  In2/1 -> AND/1
  In1/1 -> AND/2

== system merged/Tri state buffer42 ==
  In1 : Inport
  In2 : Inport  Port=2
  AND : Logic  IconShape=distinctive  AllPortsSameDT=off  OutDataTypeStr=boolean
  Out1 : Outport
  wires:
  AND/1 -> Out1/1
  In2/1 -> AND/1
  In1/1 -> AND/2

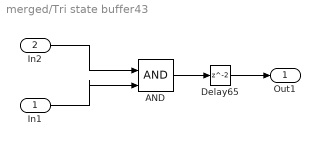
== system merged/Tri state buffer43 ==
  In1 : Inport
  In2 : Inport  Port=2
  AND : Logic  IconShape=distinctive  AllPortsSameDT=off  OutDataTypeStr=boolean
  Delay65 : Delay
  Out1 : Outport
  wires:
  In1/1 -> AND/2
  In2/1 -> AND/1
  AND/1 -> Delay65/1
  Delay65/1 -> Out1/1

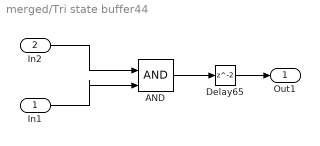
== system merged/Tri state buffer44 ==
  In1 : Inport
  In2 : Inport  Port=2
  AND : Logic  IconShape=distinctive  AllPortsSameDT=off  OutDataTypeStr=boolean
  Delay65 : Delay
  Out1 : Outport
  wires:
  In1/1 -> AND/2
  In2/1 -> AND/1
  AND/1 -> Delay65/1
  Delay65/1 -> Out1/1

== system merged/Tri state buffer45 ==
  In1 : Inport
  In2 : Inport  Port=2
  AND : Logic  IconShape=distinctive  AllPortsSameDT=off  OutDataTypeStr=boolean
  Out1 : Outport
  wires:
  AND/1 -> Out1/1
  In2/1 -> AND/1
  In1/1 -> AND/2

== system merged/Tri state buffer46 ==
  In1 : Inport
  In2 : Inport  Port=2
  AND : Logic  IconShape=distinctive  AllPortsSameDT=off  OutDataTypeStr=boolean
  Out1 : Outport
  wires:
  AND/1 -> Out1/1
  In2/1 -> AND/1
  In1/1 -> AND/2

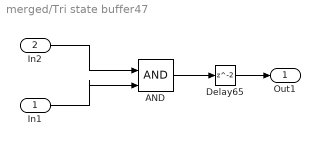
== system merged/Tri state buffer47 ==
  In1 : Inport
  In2 : Inport  Port=2
  AND : Logic  IconShape=distinctive  AllPortsSameDT=off  OutDataTypeStr=boolean
  Delay65 : Delay
  Out1 : Outport
  wires:
  In1/1 -> AND/2
  In2/1 -> AND/1
  AND/1 -> Delay65/1
  Delay65/1 -> Out1/1

== system merged/Tri state buffer48 ==
  In1 : Inport
  In2 : Inport  Port=2
  AND : Logic  IconShape=distinctive  AllPortsSameDT=off  OutDataTypeStr=boolean
  Out1 : Outport
  wires:
  In1/1 -> AND/2
  In2/1 -> AND/1
  AND/1 -> Out1/1

== system merged/Tri state buffer49 ==
  In1 : Inport
  In2 : Inport  Port=2
  AND : Logic  IconShape=distinctive  AllPortsSameDT=off  OutDataTypeStr=boolean
  Out1 : Outport
  wires:
  In1/1 -> AND/2
  In2/1 -> AND/1
  AND/1 -> Out1/1

== system merged/Tri state buffer5 ==
  In1 : Inport
  In2 : Inport  Port=2
  AND : Logic  IconShape=distinctive  AllPortsSameDT=off  OutDataTypeStr=boolean
  Out1 : Outport
  wires:
  AND/1 -> Out1/1
  In2/1 -> AND/1
  In1/1 -> AND/2

== system merged/Tri state buffer50 ==
  In1 : Inport
  In2 : Inport  Port=2
  AND : Logic  IconShape=distinctive  AllPortsSameDT=off  OutDataTypeStr=boolean
  Out1 : Outport
  wires:
  In1/1 -> AND/2
  In2/1 -> AND/1
  AND/1 -> Out1/1

== system merged/Tri state buffer51 ==
  In1 : Inport
  In2 : Inport  Port=2
  AND : Logic  IconShape=distinctive  AllPortsSameDT=off  OutDataTypeStr=boolean
  Out1 : Outport
  wires:
  In1/1 -> AND/2
  In2/1 -> AND/1
  AND/1 -> Out1/1

== system merged/Tri state buffer52 ==
  In1 : Inport
  In2 : Inport  Port=2
  AND : Logic  IconShape=distinctive  AllPortsSameDT=off  OutDataTypeStr=boolean
  Out1 : Outport
  wires:
  AND/1 -> Out1/1
  In2/1 -> AND/1
  In1/1 -> AND/2

== system merged/Tri state buffer53 ==
  In1 : Inport
  In2 : Inport  Port=2
  AND : Logic  IconShape=distinctive  AllPortsSameDT=off  OutDataTypeStr=boolean
  Out1 : Outport
  wires:
  AND/1 -> Out1/1
  In2/1 -> AND/1
  In1/1 -> AND/2

== system merged/Tri state buffer54 ==
  In1 : Inport
  In2 : Inport  Port=2
  AND : Logic  IconShape=distinctive  AllPortsSameDT=off  OutDataTypeStr=boolean
  Out1 : Outport
  wires:
  AND/1 -> Out1/1
  In2/1 -> AND/1
  In1/1 -> AND/2

== system merged/Tri state buffer55 ==
  In1 : Inport
  In2 : Inport  Port=2
  AND : Logic  IconShape=distinctive  AllPortsSameDT=off  OutDataTypeStr=boolean
  Out1 : Outport
  wires:
  AND/1 -> Out1/1
  In2/1 -> AND/1
  In1/1 -> AND/2

== system merged/Tri state buffer6 ==
  In1 : Inport
  In2 : Inport  Port=2
  AND : Logic  IconShape=distinctive  AllPortsSameDT=off  OutDataTypeStr=boolean
  Out1 : Outport
  wires:
  In1/1 -> AND/2
  In2/1 -> AND/1
  AND/1 -> Out1/1

== system merged/Tri state buffer8 ==
  In1 : Inport
  In2 : Inport  Port=2
  AND : Logic  IconShape=distinctive  AllPortsSameDT=off  OutDataTypeStr=boolean
  Out1 : Outport
  wires:
  AND/1 -> Out1/1
  In2/1 -> AND/1
  In1/1 -> AND/2

== system merged/Tri state buffer9 ==
  In1 : Inport
  In2 : Inport  Port=2
  AND : Logic  IconShape=distinctive  AllPortsSameDT=off  OutDataTypeStr=boolean
  Out1 : Outport
  wires:
  In1/1 -> AND/2
  In2/1 -> AND/1
  AND/1 -> Out1/1

== system merged/buffer ==
  In1 : Inport
  Out1 : Outport
  wires:
  In1/1 -> Out1/1

== system merged/buffer1 ==
  In1 : Inport
  Out1 : Outport
  wires:
  In1/1 -> Out1/1

== system merged/buffer10 ==
  In1 : Inport
  Out1 : Outport
  wires:
  In1/1 -> Out1/1

== system merged/buffer11 ==
  In1 : Inport
  Out1 : Outport
  wires:
  In1/1 -> Out1/1

== system merged/buffer12 ==
  In1 : Inport
  Out1 : Outport
  wires:
  In1/1 -> Out1/1

== system merged/buffer13 ==
  In1 : Inport
  Out1 : Outport
  wires:
  In1/1 -> Out1/1

== system merged/buffer14 ==
  In1 : Inport
  Out1 : Outport
  wires:
  In1/1 -> Out1/1

== system merged/buffer15 ==
  In1 : Inport
  Out1 : Outport
  wires:
  In1/1 -> Out1/1

== system merged/buffer16 ==
  In1 : Inport
  Out1 : Outport
  wires:
  In1/1 -> Out1/1

== system merged/buffer17 ==
  In1 : Inport
  Out1 : Outport
  wires:
  In1/1 -> Out1/1

== system merged/buffer18 ==
  In1 : Inport
  Out1 : Outport
  wires:
  In1/1 -> Out1/1

== system merged/buffer19 ==
  In1 : Inport
  Out1 : Outport
  wires:
  In1/1 -> Out1/1

== system merged/buffer2 ==
  In1 : Inport
  Out1 : Outport
  wires:
  In1/1 -> Out1/1

== system merged/buffer20 ==
  In1 : Inport
  Out1 : Outport
  wires:
  In1/1 -> Out1/1

== system merged/buffer21 ==
  In1 : Inport
  Out1 : Outport
  wires:
  In1/1 -> Out1/1

== system merged/buffer22 ==
  In1 : Inport
  Out1 : Outport
  wires:
  In1/1 -> Out1/1

== system merged/buffer23 ==
  In1 : Inport
  Out1 : Outport
  wires:
  In1/1 -> Out1/1

== system merged/buffer24 ==
  In1 : Inport
  Out1 : Outport
  wires:
  In1/1 -> Out1/1

== system merged/buffer25 ==
  In1 : Inport
  Out1 : Outport
  wires:
  In1/1 -> Out1/1

== system merged/buffer26 ==
  In1 : Inport
  Out1 : Outport
  wires:
  In1/1 -> Out1/1

== system merged/buffer27 ==
  In1 : Inport
  Out1 : Outport
  wires:
  In1/1 -> Out1/1

== system merged/buffer28 ==
  In1 : Inport
  Out1 : Outport
  wires:
  In1/1 -> Out1/1

== system merged/buffer29 ==
  In1 : Inport
  Out1 : Outport
  wires:
  In1/1 -> Out1/1

== system merged/buffer3 ==
  In1 : Inport
  Out1 : Outport
  wires:
  In1/1 -> Out1/1

== system merged/buffer30 ==
  In1 : Inport
  Out1 : Outport
  wires:
  In1/1 -> Out1/1

== system merged/buffer31 ==
  In1 : Inport
  Out1 : Outport
  wires:
  In1/1 -> Out1/1

== system merged/buffer4 ==
  In1 : Inport
  Out1 : Outport
  wires:
  In1/1 -> Out1/1

== system merged/buffer5 ==
  In1 : Inport
  Out1 : Outport
  wires:
  In1/1 -> Out1/1

== system merged/buffer6 ==
  In1 : Inport
  Out1 : Outport
  wires:
  In1/1 -> Out1/1

== system merged/buffer7 ==
  In1 : Inport
  Out1 : Outport
  wires:
  In1/1 -> Out1/1

== system merged/buffer8 ==
  In1 : Inport
  Out1 : Outport
  wires:
  In1/1 -> Out1/1

== system merged/buffer9 ==
  In1 : Inport
  Out1 : Outport
  wires:
  In1/1 -> Out1/1

== matlab function merged/Program Counter ==
  data: y output; clk input
function y = ring_counter(clk)
% 7-bit Ring Counter
persistent state
if isempty(state)
    state = [1 0 0 0 0 0 0]; % Initial state
end

if clk == 1
    state = circshift(state, [0 1]); % Shift right
end

y = state;

== matlab function merged/Ring Counter ==
  data: y output; clk input
function y = ring_counter(clk)
% 7-bit Ring Counter
persistent state
if isempty(state)
    state = [1 0 0 0 0 0 0]; % Initial state
end

if clk == 1
    state = circshift(state, [0 1]); % Shift right
end

y = state;
